simulink model "select_lo_mid_hi_rate"  (R2018b)
settings: Solver=VariableStepAuto  StartTime=0.0  StopTime=10.0  RelTol=1e-3
values from neighbouring files (symbols this model uses):
  roomVol = roomVol*1.15    [Setup_Code_EWASP_VC.m]
undefined symbols (not defined in the file or in its folder): ExtractRates, TempVecInKelvins
settings Model: Creator=cpp14rcj  LastModifiedBy=cpp14rcj

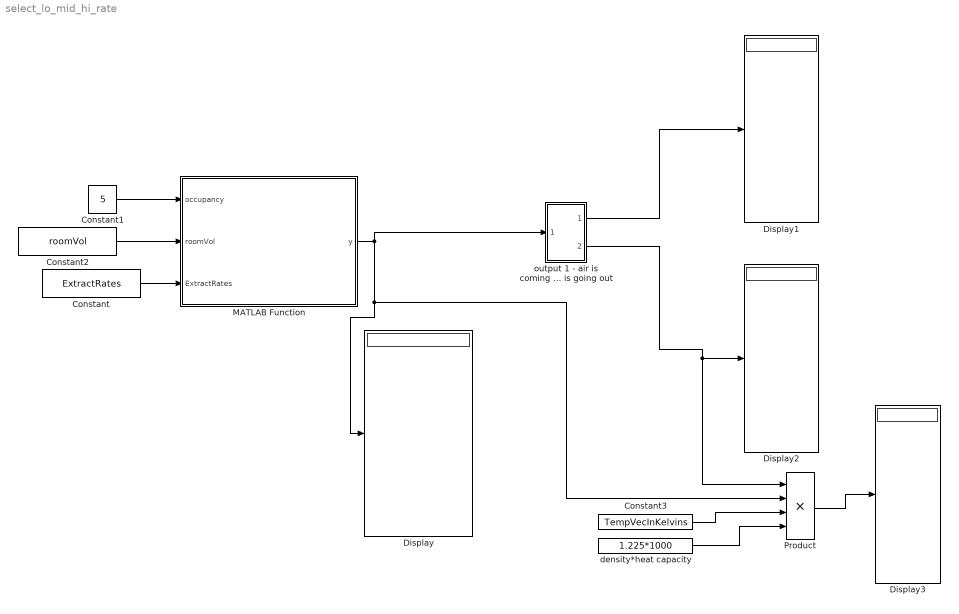
== system select_lo_mid_hi_rate ==
  " output 1 - air is coming in output 2 - air is going out" : Subsystem
  Constant : Constant  Value=ExtractRates
  Constant1 : Constant  Value=5
  Constant2 : Constant  Value=roomVol
  Constant3 : Constant  Value=TempVecInKelvins
  Display{,1..3} (4 alike) : Display
  MATLAB Function : MATLAB Function  TreatAsAtomicUnit=on
  Product : Product  Inputs=4
  density*heat capacity : Constant  Value=1.225*1000
  wires:
  Constant/1 -> MATLAB Function/3(ExtractRates)
  Constant1/1 -> MATLAB Function/1(occupancy)
  Constant2/1 -> MATLAB Function/2(roomVol)
  MATLAB Function/1(y) -> " output 1 - air is coming in output 2 - air is going out"/1(In1), Product/2, Display/1
  " output 1 - air is coming in output 2 - air is going out"/1(Out1) -> Display1/1
  " output 1 - air is coming in output 2 - air is going out"/2(Out2) -> Product/1, Display2/1
  Constant3/1 -> Product/3
  density*heat capacity/1 -> Product/4
  Product/1 -> Display3/1

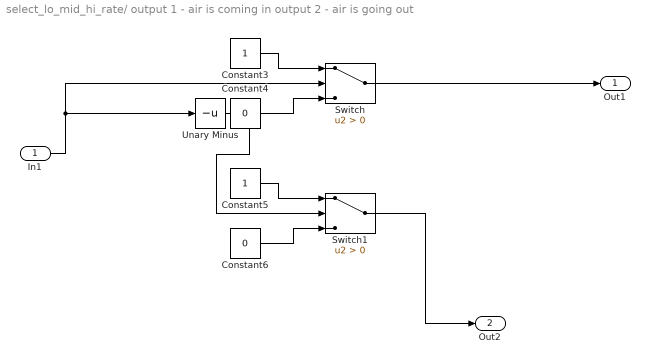
== system select_lo_mid_hi_rate/ output 1 - air is coming in output 2 - air is going out ==
  In1 : Inport
  Constant3 : Constant
  Constant4 : Constant  Value=0
  Constant5 : Constant
  Constant6 : Constant  Value=0
  Switch : Switch  Criteria=u2 > Threshold
  Switch1 : Switch  Criteria=u2 > Threshold
  Unary Minus : UnaryMinus
  Out1 : Outport
  Out2 : Outport  Port=2
  wires:
  Unary Minus/1 -> Switch1/2
  In1/1 -> Unary Minus/1, Switch/2
  Constant6/1 -> Switch1/3
  Switch1/1 -> Out2/1
  Switch/1 -> Out1/1
  Constant5/1 -> Switch1/1
  Constant4/1 -> Switch/3
  Constant3/1 -> Switch/1

== matlab function select_lo_mid_hi_rate/MATLAB Function ==
  data: occupancy input; roomVol input; y output; ExtractRates input
function y = fcn(occupancy,roomVol,ExtractRates)

if occupancy == 0 % no one is in
    
    y=ExtractRates(:,1);
    
elseif occupancy*30<sum(roomVol)*0.3 %occupancy is greater than 0, but less than that wich would require the system to be boosted byone the minimum occupied 0.3 ACR
    
    y=ExtractRates(:,2);
    
else %occupancy*30 m3/h is greater than the minimum 0.3ACR*houseVol
    
    y=ExtractRates(:,3);
    
end
